simulink model "simpark"  (R2015b)
settings: Solver=VariableStepAuto  StartTime=0.0  StopTime=100  RelTol=1e-3
values from neighbouring files (symbols this model uses):
  dir = -1    [parkfil.m]
  fi0 = Fi.signals.values(c)    [parkfil.m]
  park = 1    [parkfil.m]
  x0 = X.signals.values(c)    [parkfil.m]
  y0 = Y.signals.values(c)    [parkfil.m]
  ystep = 10    [parkfil.m]
libraries: fuzblock x2, simulink x2
settings Model: Creator=yasin_A  LastModifiedBy=yasin_A

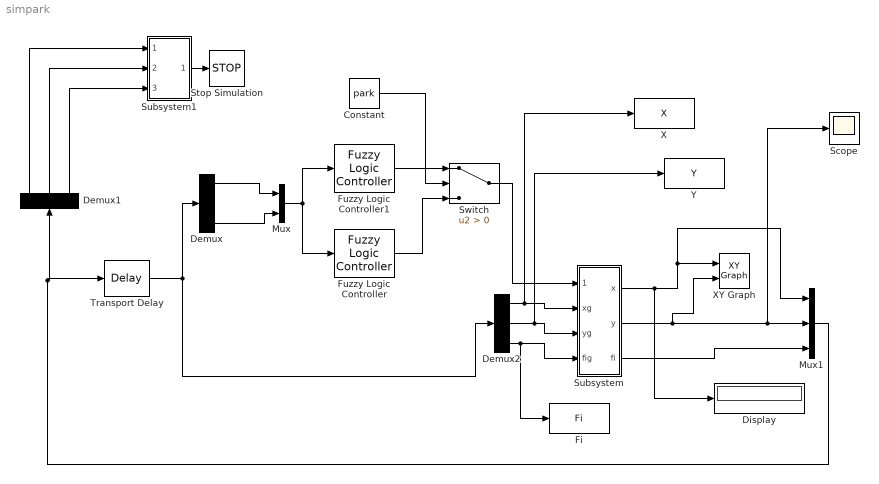
== system simpark ==
  Constant : Constant  Value=park
  Demux : Demux  Outputs=3
  Demux1 : Demux  Outputs=3
  Demux2 : Demux  Outputs=3
  Display : Display
  Fi : ToWorkspace  VariableName=Fi  SaveFormat=Structure  SampleTime=-1
  Fuzzy Logic Controller : fuzblock/Fuzzy Logic  Controller  fis='tstop.fis'
  Fuzzy Logic Controller1 : fuzblock/Fuzzy Logic  Controller  fis='tpark.fis'
  Mux : Mux  Inputs=2
  Mux1 : Mux  Inputs=3
  Scope : Scope
  Stop Simulation : Stop
  Subsystem : Subsystem
  Subsystem1 : Subsystem
  Switch : Switch  Criteria=u2 > Threshold
  Transport Delay : TransportDelay  InitialOutput=[x0 y0 fi0]
  X : ToWorkspace  VariableName=X  SaveFormat=Structure  SampleTime=-1
  XY Graph : simulink/Sinks/XY Graph  xmin=0  xmax=20  ymin=0  ymax=40  st=-1
  Y : ToWorkspace  VariableName=Y  SaveFormat=Structure  SampleTime=-1
  wires:
  Mux/1 -> Fuzzy Logic Controller/1, Fuzzy Logic Controller1/1
  Subsystem/2(y) -> XY Graph/2, Mux1/2, Scope/1
  Demux/1 -> Mux/1
  Transport Delay/1 -> Demux/1, Demux2/1
  Subsystem/3(fi) -> Mux1/3
  Demux/3 -> Mux/2
  Subsystem1/1(Out1) -> Stop Simulation/1
  Mux1/1 -> Demux1/1, Transport Delay/1
  Demux1/1 -> Subsystem1/1(In1)
  Demux1/3 -> Subsystem1/3(In2)
  Demux2/1 -> X/1, Subsystem/2(xg)
  Demux2/2 -> Y/1, Subsystem/3(yg)
  Demux2/3 -> Subsystem/4(fig), Fi/1
  Demux1/2 -> Subsystem1/2(In3)
  Subsystem/1(x) -> Display/1, Mux1/1, XY Graph/1
  Switch/1 -> Subsystem/1(teta)
  Constant/1 -> Switch/2
  Fuzzy Logic Controller/1 -> Switch/3
  Fuzzy Logic Controller1/1 -> Switch/1

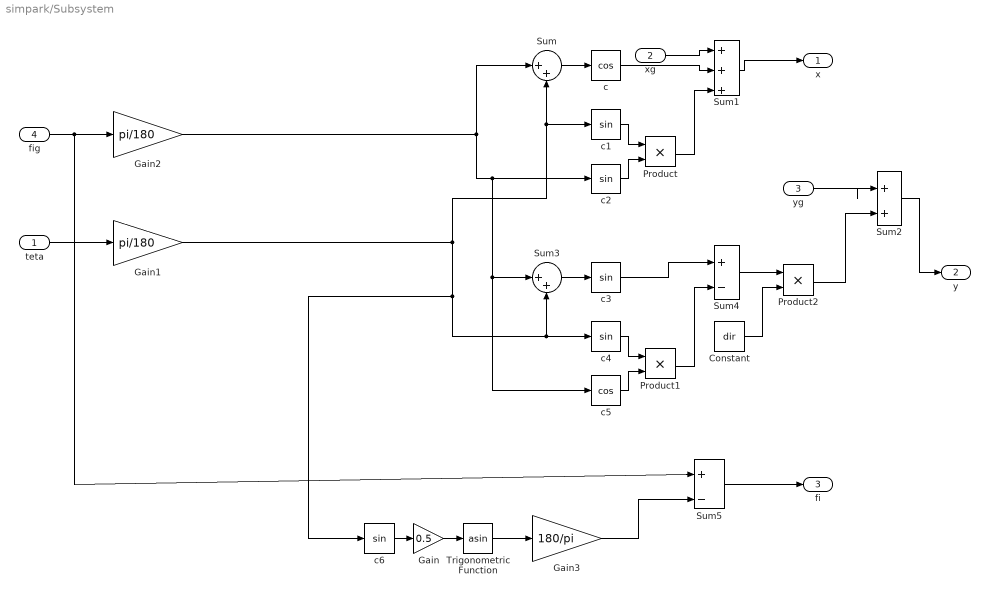
== system simpark/Subsystem ==
  teta : Inport
  xg : Inport  Port=2
  yg : Inport  Port=3
  fig : Inport  Port=4
  Constant : Constant  Value=dir
  Gain : Gain  Gain=0.5
  Gain1 : Gain  Gain=pi/180
  Gain2 : Gain  Gain=pi/180
  Gain3 : Gain  Gain=180/pi
  Product : Product
  Product1 : Product
  Product2 : Product
  Sum : Sum  Inputs=|++
  Sum1 : Sum  Inputs=|+++
  Sum2 : Sum  Inputs=|++
  Sum3 : Sum  Inputs=|++
  Sum4 : Sum  Inputs=|+-
  Sum5 : Sum  Inputs=|+-
  Trigonometric Function : Trigonometry  Operator=asin
  c : Trigonometry  Operator=cos
  c{1..4,6} (5 alike) : Trigonometry
  c5 : Trigonometry  Operator=cos
  x : Outport
  y : Outport  Port=2
  fi : Outport  Port=3
  wires:
  Sum/1 -> c/1
  Sum1/1 -> x/1
  c/1 -> Sum1/2
  c1/1 -> Product/1
  c2/1 -> Product/2
  Product/1 -> Sum1/3
  xg/1 -> Sum1/1
  Sum3/1 -> c3/1
  fig/1 -> Sum5/1, Gain2/1
  teta/1 -> Gain1/1
  c4/1 -> Product1/1
  c5/1 -> Product1/2
  Product1/1 -> Sum4/2
  Sum5/1 -> fi/1
  c6/1 -> Gain/1
  Gain/1 -> Trigonometric Function/1
  Gain1/1 -> c1/1, Sum/2, c6/1, c4/1, Sum3/2
  Gain2/1 -> c5/1, Sum3/1, c2/1, Sum/1
  Trigonometric Function/1 -> Gain3/1
  Gain3/1 -> Sum5/2
  yg/1 -> Sum2/1
  Sum4/1 -> Product2/1
  Sum2/1 -> y/1
  Product2/1 -> Sum2/2
  c3/1 -> Sum4/1
  Constant/1 -> Product2/2

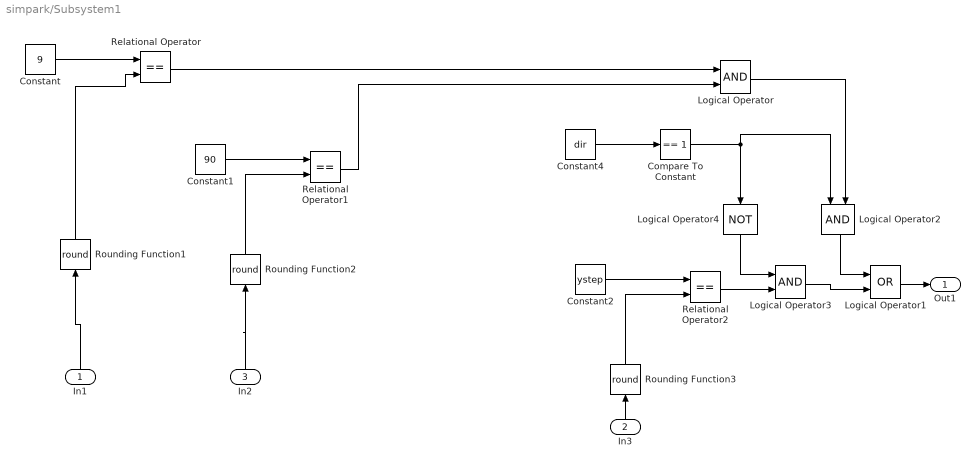
== system simpark/Subsystem1 ==
  In1 : Inport
  In3 : Inport  Port=2
  In2 : Inport  Port=3
  Compare To Constant : simulink/Logic and Bit Operations/Compare To Constant  relop===  const=1  OutDataTypeStr=boolean
  Constant : Constant  Value=9
  Constant1 : Constant  Value=90
  Constant2 : Constant  Value=ystep
  Constant4 : Constant  Value=dir
  Logical Operator : Logic  AllPortsSameDT=off  OutDataTypeStr=boolean
  Logical Operator1 : Logic  Operator=OR  AllPortsSameDT=off  OutDataTypeStr=boolean
  Logical Operator2 : Logic  AllPortsSameDT=off  OutDataTypeStr=boolean
  Logical Operator3 : Logic  AllPortsSameDT=off  OutDataTypeStr=boolean
  Logical Operator4 : Logic  Operator=NOT  AllPortsSameDT=off  OutDataTypeStr=boolean
  Relational Operator : RelationalOperator  Operator===  OutDataTypeStr=boolean
  Relational Operator1 : RelationalOperator  Operator===  OutDataTypeStr=boolean
  Relational Operator2 : RelationalOperator  Operator===  OutDataTypeStr=boolean
  Rounding Function1 : Rounding  Operator=round
  Rounding Function2 : Rounding  Operator=round
  Rounding Function3 : Rounding  Operator=round
  Out1 : Outport
  wires:
  Constant1/1 -> Relational Operator1/1
  Rounding Function2/1 -> Relational Operator1/2
  Constant/1 -> Relational Operator/1
  In2/1 -> Rounding Function2/1
  In1/1 -> Rounding Function1/1
  Rounding Function1/1 -> Relational Operator/2
  Relational Operator/1 -> Logical Operator/1
  Relational Operator1/1 -> Logical Operator/2
  Constant2/1 -> Relational Operator2/1
  Rounding Function3/1 -> Relational Operator2/2
  In3/1 -> Rounding Function3/1
  Logical Operator1/1 -> Out1/1
  Logical Operator2/1 -> Logical Operator1/1
  Logical Operator/1 -> Logical Operator2/2
  Logical Operator3/1 -> Logical Operator1/2
  Relational Operator2/1 -> Logical Operator3/2
  Logical Operator4/1 -> Logical Operator3/1
  Constant4/1 -> Compare To Constant/1
  Compare To Constant/1 -> Logical Operator2/1, Logical Operator4/1
